simulink model "book_5_6"  (R2019a)
settings: Solver=ode23t  StartTime=0.0  StopTime=0.1  FixedStep=1e-5  RelTol=1e-4  EnableMultiTasking=on
undefined symbols (not defined in the file): Ts
libraries: powerlib x8, powerlib_meascontrol x1
settings Model: Creator=umi  LastModifiedBy=Zezzid
settings DataIOCC: LimitDataPoints=on  SaveFormat=Array  ReturnWorkspaceOutputs=off
settings OptimizationCC: LifeSpan=inf
settings DebuggingCC: SolverPrmCheckMsg=warning  SFUnexpectedBacktrackingDiag=warning  SFNoUnconditionalDefaultTransitionDiag=warning  SFExecutionAtInitializationDiag=none  ArithmeticOperatorsInVariantConditions=warning
settings HardwareCC: ProdBitPerPointer=32  ProdBitPerSizeT=32  ProdBitPerPtrDiffT=32  ProdLargestAtomicFloat=None  ProdIntDivRoundTo=Undefined  ProdEndianess=Unspecified  ProdWordSize=32  ProdHWDeviceType=32-bit Generic
settings ModelReferenceCC: PropagateSignalLabelsOutOfModel=off
settings SFSimCC: SimUseLocalCustomCode=off
settings RTWCC: RTWUseLocalCustomCode=off
settings CodeAppCC: StateflowObjectComments=on
settings GRTTargetCC: TargetLangStandard=C89/C90 (ANSI)  GeneratePreprocessorConditionals=Disable all
settings ConfigComp: CovMetricSettings=dw  CovHtmlReporting=on  CovSaveCumulativeToWorkspaceVar=on  CovSaveSingleToWorkspaceVar=on  CovExternalEMLEnable=off  CovSFcnEnable=off
settings SimscapeCC: SimscapeNormalizeSystem=off

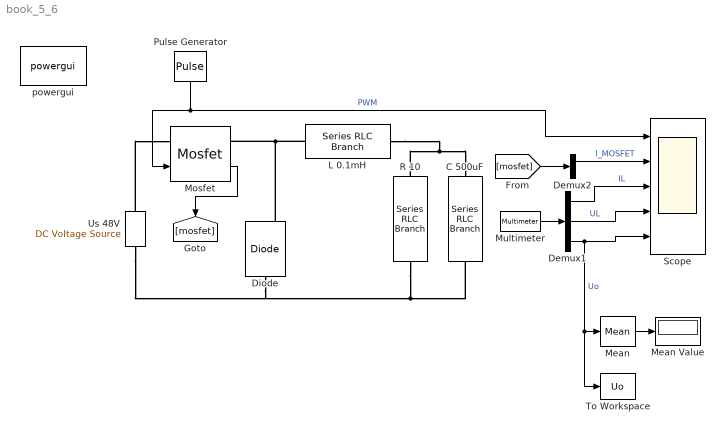
== system book_5_6 ==
  C 500uF : powerlib/Elements/Series RLC Branch  LConnTagsString=__new0  RConnTagsString=__new0  BranchType=C  Resistance=1  Inductance=0.1e-3  SetiL0=off  InitialCurrent=0  Capacitance=500e-6  Setx0=off  InitialVoltage=0  Measurements=Branch voltage
      settings: SourceProductName=Simscape Electrical
  Demux1 : Demux  Outputs=3
  Demux2 : Demux  Outputs=2
  Diode : powerlib/Power Electronics/Diode  Ron=0.001  Lon=1e-8  Vf=0.7  IC=0  UseSnubber=off  Rs=1e5  Cs=Inf  Measurements=on
      settings: SourceProductName=Simscape Electrical
  L 0.1mH : powerlib/Elements/Series RLC Branch  LConnTagsString=__new0  RConnTagsString=__new0  BranchType=L  Resistance=1  Inductance=0.1e-3  SetiL0=off  InitialCurrent=0  Capacitance=1e-6  Setx0=off  InitialVoltage=0  Measurements=Branch voltage and current
      settings: SourceProductName=Simscape Electrical
  Mean : powerlib_meascontrol/Measurements/Mean  Freq=60  Vinit=0  Ts=0
      settings: SourceProductName=Simscape Electrical
  Mean Value : Display
      settings: Format=bank
  Mosfet : powerlib/Power Electronics/Mosfet  Ron=0.1  Lon=0  Rd=0.01  Vfd=0  IC=0  Rs=1e5  Cs=inf  Measurements=on
      settings: SourceProductName=Simscape Electrical
  Multimeter : powerlib/Measurements/Multimeter  PhasorSimulation=off  OutputType=Complex  sel=[4 2 1]  L=4  Gain=[1 1 1]  yselected={'Ib: L 0.1mH','Ub: L 0.1mH','Ub: C 500uF'};  PSBOutputType=1  PSBequivalent=0  AxesSetting=[0,0.1,-100,100]  Display=0  SavedBlockNames=-11
      settings: SourceProductName=Simscape Electrical
  Pulse Generator : DiscretePulseGenerator  PulseType=Time based  Period=1e-5  PulseWidth=25
  R 10 : powerlib/Elements/Series RLC Branch  LConnTagsString=__new0  RConnTagsString=__new0  BranchType=R  Resistance=10  Inductance=1e-3  SetiL0=off  InitialCurrent=0  Capacitance=1e-6  Setx0=off  InitialVoltage=0  Measurements=Branch current
      settings: SourceProductName=Simscape Electrical
  Scope : Scope  NumInputPorts=5
  To Workspace : ToWorkspace  VariableName=Uo  SaveFormat=Timeseries  SampleTime=-1
  Us 48V : powerlib/Electrical Sources/DC Voltage Source  Amplitude=48  Measurements=None
      settings: SourceProductName=Simscape Electrical
  powergui : powerlib/powergui  Priority=1  SimulationMode=Continuous  SampleTime=Ts  frequency=60  Iterations=50  frequencyindice=0  Pbase=100e6  ErrMax=1e-4  UnitsV=kV  UnitsW=MW  buscounter=0  FunctionMessages=off  echomessages=off  EnableUseOfTLC=off  CurrentSourceSwitches=off  DisableSnubberDevices=on  DisableRonSwitches=off  DisableVfSwitches=off  DisplayEquations=off  AutomaticDiscreteSolvers=off  SolverType=Tustin/Backward Euler (TBE)  Interpol=off  ExternalGateDelay=off  methode=off  Ts=100  x0status=blocks  SPID=on  SwTol=0  HookPort=off  NonlinearTolerance=0  nMaxIteration=15  ContinueOnMaxIteration=off  RestoreLinks=warning  ResistiveCurrentMeasurement=off  Frange=[0:2:500]  Ylog=off  Xlog=on  ShowGrid=off  save=off  variable=ZData  structure=0  ZoomFFT=off  StartTime=0.0  cycles=1  DisplayStyle=1  fundamental=60  FreqAxis=off  MaxFrequency=1000  frequencyindicesteady=1  RmsSteady=1  display=off
      settings: SourceProductName=Simscape Electrical
  wires:
  Pulse Generator/1 -> Scope/1, Mosfet/1  "PWM"
  Mosfet/1 -> [mosfet]
  [mosfet] -> Demux2/1
  Demux2/1 -> Scope/2  "I_MOSFET"
  Multimeter/1 -> Demux1/1
  Demux1/1 -> Scope/3  "IL"
  Demux1/3 -> Scope/5, Mean/1, To Workspace/1  "Uo"
  Mean/1 -> Mean Value/1
  Demux1/2 -> Scope/4  "UL"
  connections:
  R 10/RConn1 -- Diode/LConn1 -- Us 48V/LConn1 -- C 500uF/RConn1
  R 10/LConn1 -- L 0.1mH/RConn1 -- C 500uF/LConn1
  Us 48V/RConn1 -- Mosfet/LConn1
  L 0.1mH/LConn1 -- Mosfet/RConn1 -- Diode/RConn1
